simulink model "smartgrids_project"  (R2019a)
settings: Solver=VariableStepAuto  StartTime=0.0  StopTime=50  RelTol=1e-3
libraries: powerlib x16, simulink_extras x3, powerlib_meascontrol x2, spsDieselMotorModel x1, re_lib x1
settings Model: Creator=nbedmuth  LastModifiedBy=nbedmuth

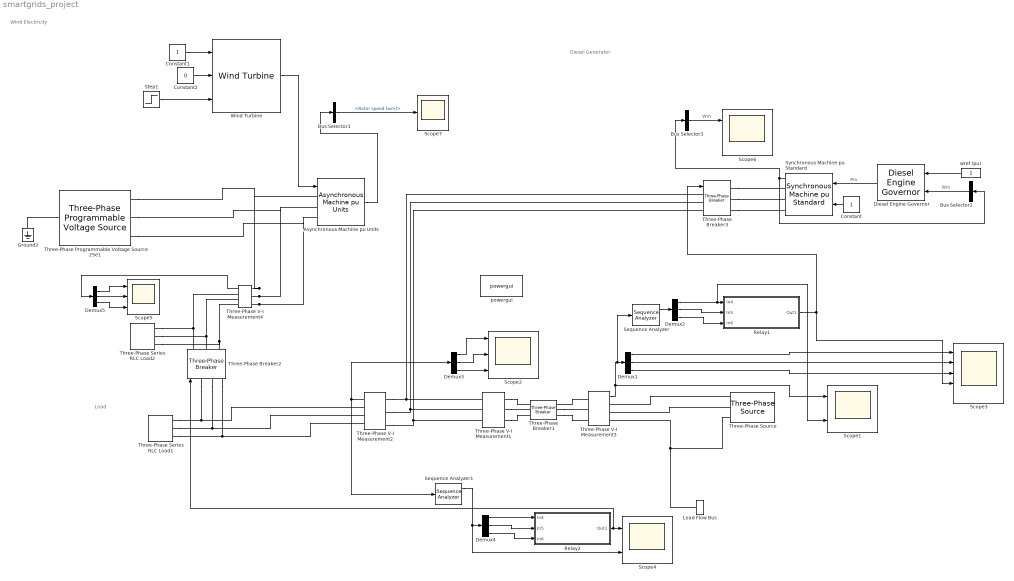
== system smartgrids_project ==
  note: Load
  note: Diesel Generator
  note: Wind Electricity
  Asynchronous Machine pu Units : powerlib/Machines/Asynchronous Machine pu Units  RotorType=Squirrel-cage  PresetModel=No  MechanicalLoad=Torque Tm  ShowDetailedParameters=on  ReferenceFrame=Rotor  Units=pu  MeasurementBus=off  NominalParameters=[1e6 575 60]  Stator=[0.01965 0.0397]  Rotor=[0.01909 0.0397]  Cage1=[0.01909 0.0397]  Cage2=[0.01909 0.0397]  Lm=1.354  Mechanical=[0.09526 0.05479 2]  PolePairs=2  InitialConditions="[ 1,0   0,0,0   0,0,0 ]"  SimulateSaturation=off  Saturation="[0.212,0.4201,0.8125,1.0979,1.4799,2.2457,3.2586,4.5763,6.4763 ;   0.5,0.7,0.9,1,1.1,1.2 ,1.3,1.4,1.5]"  LoadFlowParameters=0  TsPowergui=0  TsBlock=-1  IterativeModel=Trapezoidal non iterative  IterativeDiscreteModel=Trapezoidal non iterative  Pmec=0
      settings: SourceProductName=Simscape Electrical  SourceProductBaseCode=PS
  Bus Selector1 : BusSelector  OutputSignals=Mechanical.Rotor speed (wm)
  Bus Selector2 : BusSelector  OutputSignals="Mechanical.Rotor speed  wm  (pu)"  OutputAsBus=on
  Bus Selector3 : BusSelector  OutputSignals="Output active power   Peo (pu)"  OutputAsBus=on
  Constant : Constant
  Constant1 : Constant
  Constant2 : Constant  Value=0
  Demux{1..5} (5 alike) : Demux  Outputs=3
  Diesel Engine Governor : spsDieselMotorModel/Diesel Engine Governor  K=40  Tr=[0.01 0.02 0.2]  Ta=[0.25 0.009 0.0384]  Tlim=[0 1.1]  Td=0.2509  Pm0=0
      settings: SourceProductName=Simscape Electrical  SourceProductBaseCode=PS
  Ground2 : powerlib/Elements/Ground  LConnTagsString=a
      settings: SourceProductName=Simscape Electrical
  Load Flow Bus : powerlib/Measurements/Load Flow Bus  LConnTagsString=a  Phases=single  Connectors=on one side  ID=BUS_1  Vbase=575  Vref=1  Vangle=0  VLF=1  VLFb=1  VLFc=1  angleLF=0  angleLFb=0  angleLFc=0
      settings: SourceProductName=Simscape Electrical
  Relay1 : Subsystem
  Relay2 : Subsystem
  Scope1 : Scope  NumInputPorts=2
  Scope2 : Scope  NumInputPorts=3
  Scope3 : Scope  NumInputPorts=5
  Scope4 : Scope  NumInputPorts=2
  Scope5 : Scope  NumInputPorts=3
  Scope6 : Scope  NumInputPorts=2
  Scope7 : Scope
  Sequence Analyzer : powerlib_meascontrol/Measurements/Sequence Analyzer  Freq=60  n=1  seq=Positive Negative Zero  InInit=[1, 0]  Ts=0
      settings: SourceProductName=Simscape Electrical  SourceProductBaseCode=PS
  Sequence Analyzer1 : powerlib_meascontrol/Measurements/Sequence Analyzer  Freq=60  n=1  seq=Positive Negative Zero  InInit=[1, 0]  Ts=0
      settings: SourceProductName=Simscape Electrical  SourceProductBaseCode=PS
  Step1 : Step  Before=1  After=12  SampleTime=0
  Synchronous Machine pu Standard : powerlib/Machines/Synchronous Machine pu Standard  PresetModel=No  MechanicalLoad=Mechanical power Pm  ShowDetailedParameters=on  RotorType=Salient-pole  Units=per unit standard parameters  MeasurementBus=off  NominalParameters=[6e+05 575 60]  Reactances1=[ 1.81, 0.3, 0.23, 1.76, 0.65, 0.25, 0.15 ]  Reactances2=[1.56 0.296 0.177 1.06 0.177 0.052]  dAxisTimeConstants=Short-circuit  qAxisTimeConstants=Open-circuit  TimeConstants1="[ 4.4849  0.0681  0.1  ]"  TimeConstants2=[ 8.0, 0.03, 1.0, 0.07 ]  TimeConstants3="[  4.49  0.0681  0.0513  ]"  TimeConstants4=[ 8.0, 0.03, 0.3371, 0.0295 ]  TimeConstants5=[ 3.7, 0.05, 0.05]  TimeConstants6=[ 1.3201, 0.023, 1.0, 0.07 ]  TimeConstants7=[3.7 0.05 0.05]  TimeConstants8=[ 1.3201, 0.0231, 0.3371, 0.0295 ]  StatorResistance=0.0036  Mechanical=[1.07 0 2]  PolePairs=20  InitialConditions=[0 -90 0 0 0 0 -120 120 1]  SetSaturation=off  Saturation=[0.211 0.418 1.0 1.25 1.72 3.35; 0.25 .5 1.0 1.1 1.2 1.4]  LoadFlowParameters=[1 1000000 0 0 0]  TsPowergui=0  TsBlock=-1  IterativeModel=Trapezoidal non iterative  IterativeDiscreteModel=Trapezoidal non iterative  BusType=swing  Pref=0e6  Qref=0  Qmin=-inf  Qmax=inf  PLF=0  QLF=0
      settings: SourceProductName=Simscape Electrical
  Three-Phase Programmable Voltage Source 25e1 : powerlib/Electrical Sources/Three-Phase Programmable Voltage Source  PositiveSequence=[575 0 60]  VariationEntity=None  VariationType=Table of time-amplitude pairs  VariationTypeAlt=Step  VariationStep=0.5  VariationRate=10  VariationMagnitude=0.3  VariationFrequency=2  VariationTiming=[1 2]  VariationPhaseA=off  Amplitudes=[1 0.8 1.2 1.0]  TimeValues=[0 0.1 0.15 0.2]  HarmonicGeneration=off  HarmonicA=[3 0.2 -25 0]  HarmonicB=[2 0.15 35 2]  Timing="[0.05  3]"  BusType=PV  Pref=0  Qref=0  Qmin=-inf  Qmax=inf
      settings: SourceProductName=Simscape Electrical
  Three-Phase Series RLC Load1 : powerlib/Elements/Three-Phase Series RLC Load  LConnTagsString=A|B|C  Configuration=Y (grounded)  NominalVoltage=575  Vabc=[1e3 1e3 1e3]  Vabcp=[1e3 1e3 1e3]  NominalFrequency=60  UnbalancedPower=off  ActivePower=10e3  InductivePower=0  CapacitivePower=0  Pabc=[10e3 9e3 11e3]  QLabc=[100 90 110]  QCabc=[100 90 110]  Pabcp=[10e3 9e3 11e3]  QLabcp=[100 90 110]  QCabcp=[100 90 110]  Measurements=None  LoadType=constant Z
      settings: SourceProductName=Simscape Electrical
  Three-Phase Series RLC Load2 : powerlib/Elements/Three-Phase Series RLC Load  LConnTagsString=A|B|C  Configuration=Y (grounded)  NominalVoltage=575  Vabc=[1e3 1e3 1e3]  Vabcp=[1e3 1e3 1e3]  NominalFrequency=60  UnbalancedPower=off  ActivePower=0  InductivePower=10000  CapacitivePower=0  Pabc=[10e3 9e3 11e3]  QLabc=[100 90 110]  QCabc=[100 90 110]  Pabcp=[10e3 9e3 11e3]  QLabcp=[100 90 110]  QCabcp=[100 90 110]  Measurements=None  LoadType=constant Z
      settings: SourceProductName=Simscape Electrical
  Three-Phase V-I Measurement1 : powerlib/Measurements/Three-Phase V-I Measurement  VoltageMeasurement=no  SetLabelV=off  LabelV=Vabc  Vpu=off  VpuLL=off  CurrentMeasurement=no  SetLabelI=off  LabelI=Iabc  Ipu=off  Pbase=100e6  Vbase=500e3  OutputType=Magnitude  PhasorSimulation=off  PSBequivalent=0
      settings: SourceProductName=Simscape Electrical
  Three-Phase V-I Measurement2 : powerlib/Measurements/Three-Phase V-I Measurement  VoltageMeasurement=phase-to-phase  SetLabelV=off  LabelV=Vabc  Vpu=off  VpuLL=off  CurrentMeasurement=no  SetLabelI=off  LabelI=Iabc  Ipu=off  Pbase=100e6  Vbase=500e3  OutputType=Magnitude  PhasorSimulation=off  PSBequivalent=0
      settings: SourceProductName=Simscape Electrical
  Three-Phase V-I Measurement3 : powerlib/Measurements/Three-Phase V-I Measurement  VoltageMeasurement=no  SetLabelV=off  LabelV=Vabc  Vpu=off  VpuLL=off  CurrentMeasurement=yes  SetLabelI=off  LabelI=Iabc  Ipu=off  Pbase=100e6  Vbase=500e3  OutputType=Complex  PhasorSimulation=on  PSBequivalent=0
      settings: SourceProductName=Simscape Electrical
  Three-Phase V-I Measurement4 : powerlib/Measurements/Three-Phase V-I Measurement  VoltageMeasurement=no  SetLabelV=off  LabelV=Vabc  Vpu=off  VpuLL=off  CurrentMeasurement=yes  SetLabelI=off  LabelI=Iabc  Ipu=off  Pbase=100e6  Vbase=500e3  OutputType=Magnitude  PhasorSimulation=off  PSBequivalent=0
      settings: SourceProductName=Simscape Electrical
  Three-Phase Breaker1 : powerlib/Elements/Three-Phase Breaker  InitialState=closed  SwitchA=on  SwitchB=on  SwitchC=on  SwitchTimes=2.1  External=off  BreakerResistance=.01  SnubberResistance=1e6  SnubberCapacitance=inf  Measurements=None
      settings: SourceProductName=Simscape Electrical
  Three-Phase Breaker2 : powerlib/Elements/Three-Phase Breaker  InitialState=open  SwitchA=on  SwitchB=on  SwitchC=on  SwitchTimes="[2.2  5]"  External=on  BreakerResistance=0.01  SnubberResistance=1e6  SnubberCapacitance=inf  Measurements=None
      settings: SourceProductName=Simscape Electrical
  Three-Phase Breaker3 : powerlib/Elements/Three-Phase Breaker  InitialState=open  SwitchA=on  SwitchB=on  SwitchC=on  SwitchTimes="[2.2  5]"  External=on  BreakerResistance=0.01  SnubberResistance=1e6  SnubberCapacitance=inf  Measurements=None
      settings: SourceProductName=Simscape Electrical
  Three-Phase Source : powerlib/Electrical Sources/Three-Phase Source  InternalConnection=Yg  VoltagePhases=off  Voltage=575  PhaseAngle=10.4604  Voltage_phases=[25e3 25e3 25e3]/sqrt(3)  PhaseAngles_phases=[0 -120 +120]  Frequency=60  NonIdealSource=on  SpecifyImpedance=off  Resistance=0.8929  Inductance=16.58e-3  ShortCircuitLevel=100e6  BaseVoltage=25e3  XRratio=7  BusType=swing  Pref=10e3  Qref=0  Prefabc=[10e3, 10e3, 10e3]  Qrefabc=[0, 0, 0]  Qmin=-inf  Qmax=inf
      settings: SourceProductName=Simscape Electrical
  Wind Turbine : re_lib/Wind Generation/Wind Turbine  Pnom=1.5e6  Pelec_base=1.5e6/0.9  wind_base=12  P_wind_base=0.73  speed_nom=1.2  pitch_angle=0  c1_c6="[0.51763          116          0.4            5           21     0.006795]"  cp_nom=0.48  lambda_nom=8.1
      settings: SourceProductName=Simscape Electrical  SourceProductBaseCode=PS
  powergui : powerlib/powergui  Priority=1  SimulationMode=Continuous  SampleTime=50e-6  frequency=60  Iterations=50  frequencyindice=60  Pbase=10e6  ErrMax=0.0001  UnitsV=kV  UnitsW=MW  buscounter=0  FunctionMessages=off  echomessages=off  EnableUseOfTLC=off  CurrentSourceSwitches=off  DisableSnubberDevices=off  DisableRonSwitches=off  DisableVfSwitches=off  DisplayEquations=off  AutomaticDiscreteSolvers=off  SolverType=Tustin/Backward Euler (TBE)  Interpol=off  ExternalGateDelay=off  methode=off  Ts=100  x0status=blocks  SPID=on  SwTol=0  HookPort=off  NonlinearTolerance=0  nMaxIteration=15  ContinueOnMaxIteration=off  RestoreLinks=warning  ResistiveCurrentMeasurement=off  Frange=[0:2:500]  Ylog=off  Xlog=on  ShowGrid=off  save=off  variable=ZData  structure=0  ZoomFFT=off  StartTime=0.0  cycles=1  DisplayStyle=1  fundamental=60  FreqAxis=off  MaxFrequency=1000  frequencyindicesteady=1  RmsSteady=1  display=off
      settings: SourceProductName=Simscape Electrical
  wref (pu) : Constant
  wires:
  wref (pu)/1 -> Diesel Engine Governor/1
  Bus Selector2/1 -> Diesel Engine Governor/2  "Wm"
  Constant/1 -> Synchronous Machine pu Standard/2
  Demux1/1 -> Scope3/1
  Synchronous Machine pu Standard/1 -> Bus Selector2/1, Bus Selector3/1
  Demux1/2 -> Scope3/2
  Demux1/3 -> Scope3/3
  Diesel Engine Governor/1 -> Synchronous Machine pu Standard/1  "Pm"
  Three-Phase V-I Measurement3/1 -> Scope1/1, Sequence Analyzer/1, Demux1/1
  Relay1/1(Out1) -> Scope3/4, Three-Phase Breaker3/1
  Sequence Analyzer/1 -> Demux2/1
  Demux2/1 -> Scope1/2, Relay1/1(In4)
  Demux2/2 -> Relay1/2(In5)
  Demux2/3 -> Relay1/3(In6)
  Demux3/1 -> Scope2/1
  Demux3/2 -> Scope2/2
  Demux3/3 -> Scope2/3
  Demux4/2 -> Relay2/2(In5)
  Demux4/1 -> Relay2/1(In4)
  Sequence Analyzer1/1 -> Scope4/2, Demux4/1
  Demux4/3 -> Relay2/3(In6)
  Relay2/1(Out1) -> Three-Phase Breaker2/1, Scope4/1
  Three-Phase V-I Measurement2/1 -> Sequence Analyzer1/1, Demux3/1
  Demux5/1 -> Scope5/1
  Asynchronous Machine pu Units/1 -> Bus Selector1/1
  Demux5/2 -> Scope5/2
  Three-Phase V-I Measurement4/1 -> Demux5/1
  Bus Selector1/1 -> Scope7/1  "<Rotor speed (wm)>"
  Step1/1 -> Wind Turbine/3
  Demux5/3 -> Scope5/3
  Constant1/1 -> Wind Turbine/1
  Constant2/1 -> Wind Turbine/2
  Bus Selector3/1 -> Scope6/1  "Wm"
  Wind Turbine/1 -> Asynchronous Machine pu Units/1
  connections:
  Load Flow Bus/LConn1 -- Three-Phase V-I Measurement3/RConn3 -- Three-Phase Source/RConn3
  Three-Phase Breaker3/RConn3 -- Synchronous Machine pu Standard/RConn3
  Three-Phase Breaker3/RConn1 -- Synchronous Machine pu Standard/RConn1
  Three-Phase Breaker3/RConn2 -- Synchronous Machine pu Standard/RConn2
  Three-Phase V-I Measurement3/LConn1 -- Three-Phase Breaker1/RConn1
  Three-Phase Breaker1/RConn3 -- Three-Phase V-I Measurement3/LConn3
  Three-Phase Breaker1/RConn2 -- Three-Phase V-I Measurement3/LConn2
  Three-Phase Breaker3/LConn1 -- Three-Phase V-I Measurement2/LConn1 -- Three-Phase V-I Measurement1/RConn1
  Three-Phase Breaker3/LConn2 -- Three-Phase V-I Measurement2/LConn2 -- Three-Phase V-I Measurement1/RConn2
  Three-Phase Breaker3/LConn3 -- Three-Phase V-I Measurement2/LConn3 -- Three-Phase V-I Measurement1/RConn3
  Three-Phase V-I Measurement1/LConn1 -- Three-Phase Breaker1/LConn1
  Three-Phase V-I Measurement1/LConn2 -- Three-Phase Breaker1/LConn2
  Three-Phase V-I Measurement1/LConn3 -- Three-Phase Breaker1/LConn3
  Three-Phase Source/RConn1 -- Three-Phase V-I Measurement3/RConn1
  Three-Phase Source/RConn2 -- Three-Phase V-I Measurement3/RConn2
  Three-Phase Series RLC Load1/LConn1 -- Three-Phase V-I Measurement2/RConn1 -- Three-Phase Breaker2/LConn1
  Three-Phase Series RLC Load1/LConn2 -- Three-Phase V-I Measurement2/RConn2 -- Three-Phase Breaker2/LConn2
  Three-Phase Series RLC Load1/LConn3 -- Three-Phase Breaker2/LConn3 -- Three-Phase V-I Measurement2/RConn3
  Three-Phase V-I Measurement4/LConn2 -- Asynchronous Machine pu Units/LConn2 -- Three-Phase Programmable Voltage Source 25e1/RConn2
  Three-Phase V-I Measurement4/LConn1 -- Asynchronous Machine pu Units/LConn1 -- Three-Phase Programmable Voltage Source 25e1/RConn1
  Three-Phase V-I Measurement4/LConn3 -- Asynchronous Machine pu Units/LConn3 -- Three-Phase Programmable Voltage Source 25e1/RConn3
  Three-Phase Breaker2/RConn1 -- Three-Phase V-I Measurement4/RConn1 -- Three-Phase Series RLC Load2/LConn1
  Three-Phase Breaker2/RConn2 -- Three-Phase V-I Measurement4/RConn2 -- Three-Phase Series RLC Load2/LConn2
  Three-Phase V-I Measurement4/RConn3 -- Three-Phase Series RLC Load2/LConn3 -- Three-Phase Breaker2/RConn3
  Three-Phase Programmable Voltage Source 25e1/LConn1 -- Ground2/LConn1

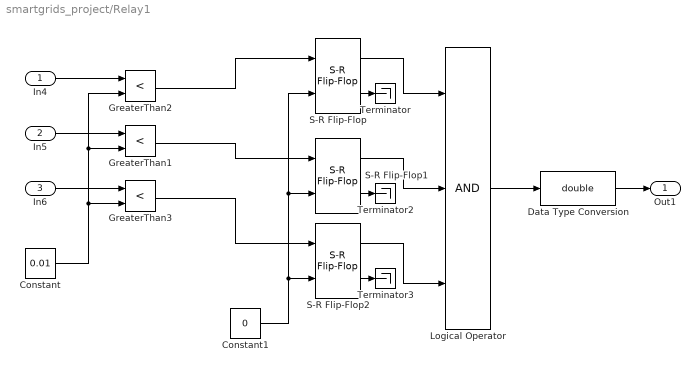
== system smartgrids_project/Relay1 ==
  In4 : Inport
  In5 : Inport  Port=2
  In6 : Inport  Port=3
  Constant : Constant  Value=0.01
  Constant1 : Constant  Value=0  OutDataTypeStr=boolean
  Data Type Conversion : DataTypeConversion  OutDataTypeStr=double
  GreaterThan1 : RelationalOperator  Operator=<  OutDataTypeStr=boolean  RndMeth=Simplest
  GreaterThan2 : RelationalOperator  Operator=<  OutDataTypeStr=boolean  RndMeth=Simplest
  GreaterThan3 : RelationalOperator  Operator=<  OutDataTypeStr=boolean  RndMeth=Simplest
  Logical Operator : Logic  Inputs=3  AllPortsSameDT=off  OutDataTypeStr=boolean
  S-R Flip-Flop : simulink_extras/Flip Flops/S-R Flip-Flop  initial_condition=0
  S-R Flip-Flop1 : simulink_extras/Flip Flops/S-R Flip-Flop  initial_condition=0
  S-R Flip-Flop2 : simulink_extras/Flip Flops/S-R Flip-Flop  initial_condition=0
  Terminator : Terminator
  Terminator2 : Terminator
  Terminator3 : Terminator
  Out1 : Outport
  wires:
  In4/1 -> GreaterThan2/1
  GreaterThan2/1 -> S-R Flip-Flop/1
  GreaterThan3/1 -> S-R Flip-Flop2/1
  GreaterThan1/1 -> S-R Flip-Flop1/1
  In5/1 -> GreaterThan1/1
  Constant/1 -> GreaterThan3/2, GreaterThan1/2, GreaterThan2/2
  In6/1 -> GreaterThan3/1
  Constant1/1 -> S-R Flip-Flop2/2, S-R Flip-Flop1/2, S-R Flip-Flop/2
  S-R Flip-Flop/1 -> Logical Operator/1
  S-R Flip-Flop1/1 -> Logical Operator/2
  S-R Flip-Flop2/1 -> Logical Operator/3
  Logical Operator/1 -> Data Type Conversion/1
  Data Type Conversion/1 -> Out1/1
  S-R Flip-Flop/2 -> Terminator/1
  S-R Flip-Flop1/2 -> Terminator2/1
  S-R Flip-Flop2/2 -> Terminator3/1

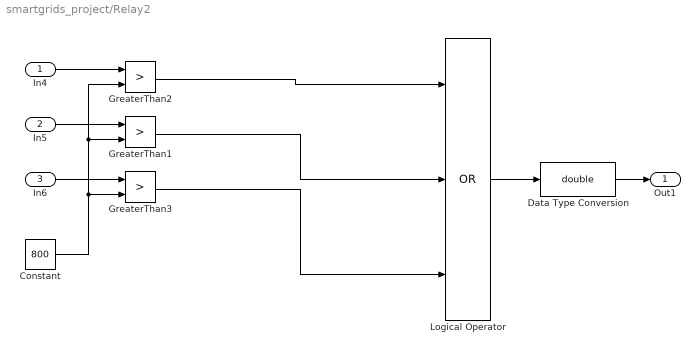
== system smartgrids_project/Relay2 ==
  In4 : Inport
  In5 : Inport  Port=2
  In6 : Inport  Port=3
  Constant : Constant  Value=800
  Data Type Conversion : DataTypeConversion  OutDataTypeStr=double
  GreaterThan1 : RelationalOperator  Operator=>  OutDataTypeStr=boolean  RndMeth=Simplest
  GreaterThan2 : RelationalOperator  Operator=>  OutDataTypeStr=boolean  RndMeth=Simplest
  GreaterThan3 : RelationalOperator  Operator=>  OutDataTypeStr=boolean  RndMeth=Simplest
  Logical Operator : Logic  Operator=OR  Inputs=3  AllPortsSameDT=off  OutDataTypeStr=boolean
  Out1 : Outport
  wires:
  In4/1 -> GreaterThan2/1
  In5/1 -> GreaterThan1/1
  Constant/1 -> GreaterThan3/2, GreaterThan1/2, GreaterThan2/2
  In6/1 -> GreaterThan3/1
  Logical Operator/1 -> Data Type Conversion/1
  Data Type Conversion/1 -> Out1/1
  GreaterThan2/1 -> Logical Operator/1
  GreaterThan1/1 -> Logical Operator/2
  GreaterThan3/1 -> Logical Operator/3
